simulink model "estimacion_ganancias"  (R2016a)
settings: Solver=ode15s  StartTime=0.0  StopTime=0.4  MaxStep=0.01  RelTol=1e-4
libraries: simulink x1
settings Model: Creator=Matias  LastModifiedBy=Matias
settings DataIOCC: LimitDataPoints=on  SaveOutput=off  SaveTime=off
settings OptimizationCC: ExpressionDepthLimit=2147483647  LifeSpan=1
settings DebuggingCC: UnderspecifiedInitializationDetection=Classic  MergeDetectMultiDrivingBlocksExec=none  FcnCallInpInsideContextMsg=EnableAllAsWarning  AllowSymbolicDim=off  StateNameClashWarn=warning
settings GRTTargetCC: CombineOutputUpdateFcns=off  GRTInterface=on

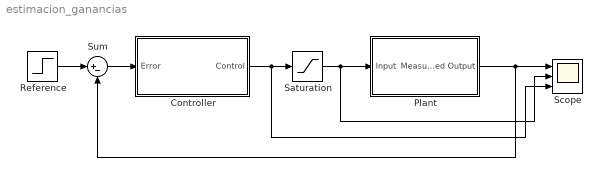
== system estimacion_ganancias ==
  Controller : Subsystem
  Plant : Subsystem
  Reference : Step  Time=0  After=2000  SampleTime=0
  Saturation : Saturate  UpperLimit=255  LowerLimit=0
  Scope : Scope  NumInputPorts=3
  Sum : Sum  Inputs=|+-
  wires:
  Reference/1 -> Sum/1
  Sum/1 -> Controller/1(Error)
  Plant/1(Measured Output) -> Sum/2, Scope/1
  Controller/1(Control) -> Scope/3, Saturation/1
  Saturation/1 -> Scope/2, Plant/1(Input)

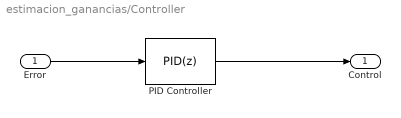
== system estimacion_ganancias/Controller ==
  Error : Inport
  PID Controller : simulink/Continuous/PID Controller  Controller=PID  TimeDomain=Discrete-time  SampleTime=0.02  IntegratorMethod=Forward Euler  FilterMethod=Backward Euler  Form=Ideal  UseFilter=on  ControllerParametersSource=internal  P=0.15  I=20  D=0  N=20  InitialConditionSource=internal  InitialConditionForIntegrator=0  InitialConditionForFilter=0  ExternalReset=none  LimitOutput=off  UpperSaturationLimit=inf  LowerSaturationLimit=-inf  LinearizeAsGain=on  AntiWindupMode=none  Kb=1  TrackingMode=off  Kt=1  PParamMin=[]  PParamMax=[]  IParamMin=[]  IParamMax=[]  DParamMin=[]  DParamMax=[]  NParamMin=[]  NParamMax=[]  KbParamMin=[]  KbParamMax=[]  KtParamMin=[]  KtParamMax=[]  POutMin=[]  POutMax=[]  IOutMin=[]  IOutMax=[]  DOutMin=[]  DOutMax=[]  NOutMin=[]  NOutMax=[]  KbOutMin=[]  KbOutMax=[]  KtOutMin=[]  KtOutMax=[]  IntegratorOutMin=[]  IntegratorOutMax=[]  FilterOutMin=[]  FilterOutMax=[]  SumOutMin=[]  SumOutMax=[]  SumI1OutMin=[]  SumI1OutMax=[]  SumI2OutMin=[]  SumI2OutMax=[]  SumI3OutMin=[]  SumI3OutMax=[]  SumDOutMin=[]  SumDOutMax=[]  SaturationOutMin=[]  SaturationOutMax=[]  IntegratorContinuousStateAttributes=''  IntegratorStateMustResolveToSignalObject=off  IntegratorRTWStateStorageClass=Auto  FilterContinuousStateAttributes=''  FilterStateMustResolveToSignalObject=off  FilterRTWStateStorageClass=Auto  DifferentiatorICPrevScaledInput=0  DifferentiatorOutMin=[]  DifferentiatorOutMax=[]
  Control : Outport
  wires:
  Error/1 -> PID Controller/1
  PID Controller/1 -> Control/1

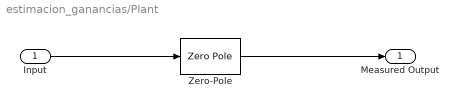
== system estimacion_ganancias/Plant ==
  Input : Inport
  Zero-Pole : ZeroPole  Zeros=[]  Poles=[-30.8]  Gain=[423.6]
  Measured Output : Outport
  wires:
  Zero-Pole/1 -> Measured Output/1
  Input/1 -> Zero-Pole/1
